simulink model "phasevocoder"  (R2020b)
settings: Solver=FixedStepDiscrete  StartTime=0.0  StopTime=4  RelTol=1e-3
values from neighbouring files (symbols this model uses):
  AnalysisHopSize = 512    [phasevocoder.mat]
  SynthesisHopSize = 512    [phasevocoder.mat]
  WindowSize = 2048    [phasevocoder.mat]
libraries: dspmtrx3 x4, dspvision x2, dspxfrm3 x2, dspsigops x2, dspsnks4 x1
settings Model: Creator=Andrea Gaetani  LastModifiedBy=Andrea Gaetani

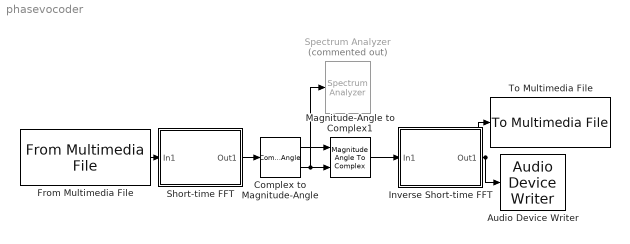
== system phasevocoder ==
  Audio Device Writer : dspsnks4/Audio Device Writer  Driver=DirectSound  Device=Default  InheritSampleRate=on  SampleRate=44100  BitDepth=16-bit integer  BufferSize=4096  NumBuffers=10  DefaultOutputChannelMapping=on  OutputChannelMapping=1:2  OutputNumUnderrunSamples=off  DriverIdx=1  DeviceWarnFlag=''
  Complex to Magnitude-Angle : ComplexToMagnitudeAngle
  From Multimedia File : dspvision/From Multimedia File  inputFilename=C:\Users\andre\Desktop\Tesina analisi dei segnali\giveloveabadname.wav  readRange=[1 Inf]  loop=on  numPlays=inf  outputStreams=Audio only  videoDataType=single  audioDataType=double  inheritSampleTime=on  userDefinedSampleTime=1/30  noAudioOutput=off  isIntensityVideo=off  fourcc=RGB  colorVideoFormat=Separate color signals  outputEOF=off  dataOrg=Column-major  audioFrameSize=1024  computeAudioFrameSize=off  outSamplingMode=Sample based
  Inverse Short-time FFT : Subsystem
      mask Display: disp('IST-FFT')
  Magnitude-Angle to Complex1 : MagnitudeAngleToComplex
  Short-time FFT : Subsystem
      mask Display: disp('ST-FFT')
  Spectrum Analyzer : SpectrumAnalyzer  Commented=on  IsFrequencyInputMode=1
  To Multimedia File : dspvision/To Multimedia File  outputFilename=C:\Users\andre\Desktop\output.wav  streamSelection=Audio only  videoCompressor=None (uncompressed)  audioCompressor=None (uncompressed)  imagePorts=Separate color signals  fileType=WAV  audioDatatype=16-bit integer  fourcc=RGB  videoQuality=75  mj2000CompFactor=10
  wires:
  Magnitude-Angle to Complex1/1 -> Inverse Short-time FFT/1(In1)
  Complex to Magnitude-Angle/1 -> Magnitude-Angle to Complex1/1
  Short-time FFT/1(Out1) -> Complex to Magnitude-Angle/1
  Inverse Short-time FFT/1(Out1) -> To Multimedia File/1, Audio Device Writer/1
  From Multimedia File/1 -> Short-time FFT/1(In1)
  Complex to Magnitude-Angle/2 -> Spectrum Analyzer/1, Magnitude-Angle to Complex1/2

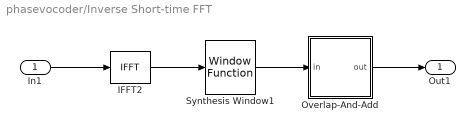
== system phasevocoder/Inverse Short-time FFT ==
  In1 : Inport
  IFFT2 : dspxfrm3/IFFT  FFTImplementation=Auto  CompMethod=Table lookup  TableOpt=HYBRID  TableOptActive=Speed  BitRevOrder=off  cs_in=on  Normalize=on  InheritFFTLength=on  FFTLength=64  WrapInput=on  mode=Complex  outSamplingMode=Sample based  roundingMode=Floor  overflowMode=off  firstCoeffMode=User-defined  firstCoeffWordLength=16  firstCoeffFracLength=15  firstCoeffDataTypeStr=fixdt(1,16)  firstCoeffLastDataTypeStr=fixdt(1,16)  accumDataTypeStr=Inherit: Same as product output  accumLastDataTypeStr=Inherit: Same as product output  outputMin=[]  outputMax=[]
      settings: SourceProductName=DSP System Toolbox
  Overlap-And-Add : Subsystem  mask(Overlap-And-Add){L=SynthesisHopSize}
      mask prompts: L "Number of new points in each frame"
      mask help: Performs overlap-and-add on the input signal. Disjoint frames of the input signal are overlapped with each other for a specified number of points and summed.
      mask Display: disp('Overlap\nAnd\nAdd')
  Synthesis Window1 : dspsigops/Window Function  winmode=Apply window to input  wintype=Hanning  sampmode=Continuous  samptime=1  N=64  Rs=50  beta=10  winsamp=Periodic  UserWindow=hamming  OptParams=off  UserParams={1.0}  dataType=double  isSigned=on  wordLen=16  udDataType=sfix(16)  fracBitsMode=Best precision  numFracBits=15  roundingMode=Floor  overflowMode=off  numSidelobes=4  sidelobeLevel=-30
      settings: SourceProductName=DSP System Toolbox
  Out1 : Outport  VectorParamsAs1DForOutWhenUnconnected=off
  wires:
  IFFT2/1 -> Synthesis Window1/1
  In1/1 -> IFFT2/1
  Synthesis Window1/1 -> Overlap-And-Add/1(in)
  Overlap-And-Add/1(out) -> Out1/1

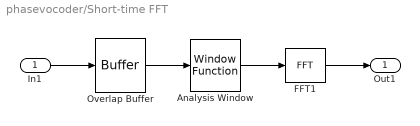
== system phasevocoder/Short-time FFT ==
  In1 : Inport
  Analysis Window : dspsigops/Window Function  winmode=Apply window to input  wintype=Hanning  sampmode=Continuous  samptime=1  N=64  Rs=50  beta=10  winsamp=Periodic  UserWindow=hamming  OptParams=off  UserParams={1.0}  dataType=double  isSigned=on  wordLen=16  udDataType=sfix(16)  fracBitsMode=Best precision  numFracBits=15  roundingMode=Floor  overflowMode=off  numSidelobes=4  sidelobeLevel=-30
      settings: SourceProductName=DSP System Toolbox
  FFT1 : dspxfrm3/FFT  FFTImplementation=Auto  CompMethod=Table lookup  TableOpt=NEW  TableOptActive=Speed  BitRevOrder=off  Normalize=off  InheritFFTLength=on  FFTLength=64  WrapInput=on  roundingMode=Floor  overflowMode=off  firstCoeffMode=Specify word length  firstCoeffWordLength=16  firstCoeffFracLength=15  firstCoeffDataTypeStr=fixdt(1,16)  firstCoeffLastDataTypeStr=fixdt(1,16)  accumDataTypeStr=Inherit: Same as product output  accumLastDataTypeStr=Inherit: Same as product output  outputMin=[]  outputMax=[]
  Overlap Buffer : Buffer  N=WindowSize  V=WindowSize-AnalysisHopSize  OutputFrames=off
  Out1 : Outport  VectorParamsAs1DForOutWhenUnconnected=off
  wires:
  Overlap Buffer/1 -> Analysis Window/1
  FFT1/1 -> Out1/1
  In1/1 -> Overlap Buffer/1
  Analysis Window/1 -> FFT1/1

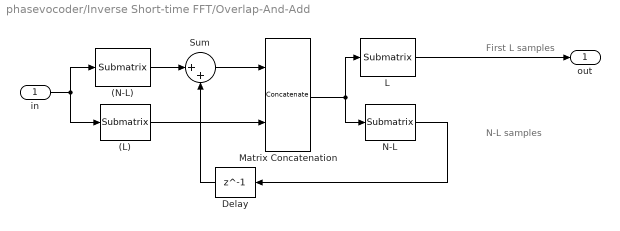
== system phasevocoder/Inverse Short-time FFT/Overlap-And-Add ==
  note: First L samples
  note: N-L samples
  in : Inport
  (L) : dspmtrx3/Submatrix  RowSpan=Range of rows  RowStartMode=Offset from last  RowStartIndex=L-1  RowEndMode=Last  RowEndIndex=1  ColSpan=All columns  ColStartMode=First  ColStartIndex=1  ColEndMode=Last  ColEndIndex=1
  (N-L) : dspmtrx3/Submatrix  RowSpan=Range of rows  RowStartMode=First  RowStartIndex=1  RowEndMode=Offset from last  RowEndIndex=L  ColSpan=All columns  ColStartMode=First  ColStartIndex=1  ColEndMode=Last  ColEndIndex=1
  Delay : Delay  DelayLength=1  InitialCondition=0
  L : dspmtrx3/Submatrix  RowSpan=Range of rows  RowStartMode=First  RowStartIndex=1  RowEndMode=Index  RowEndIndex=L  ColSpan=All columns  ColStartMode=First  ColStartIndex=1  ColEndMode=Last  ColEndIndex=1
  Matrix Concatenation : Concatenate  Mode=Multidimensional array
  N-L : dspmtrx3/Submatrix  RowSpan=Range of rows  RowStartMode=Index  RowStartIndex=L+1  RowEndMode=Last  RowEndIndex=1  ColSpan=All columns  ColStartMode=First  ColStartIndex=1  ColEndMode=Last  ColEndIndex=1
  Sum : Sum  Inputs=|++  InputSameDT=on  SaturateOnIntegerOverflow=on  OutDataTypeStr=Inherit: Same as first input
  out : Outport  VectorParamsAs1DForOutWhenUnconnected=off
  wires:
  L/1 -> out/1
  Sum/1 -> Matrix Concatenation/1
  (N-L)/1 -> Sum/1
  Delay/1 -> Sum/2
  (L)/1 -> Matrix Concatenation/2
  Matrix Concatenation/1 -> L/1, N-L/1
  in/1 -> (L)/1, (N-L)/1
  N-L/1 -> Delay/1
